simulink model "problem5"  (R2020b)
settings: Solver=VariableStepAuto  StartTime=0.0  StopTime=10.0  RelTol=1e-3
settings Model: Creator=Sourav Kumar  LastModifiedBy=Sourav Kumar

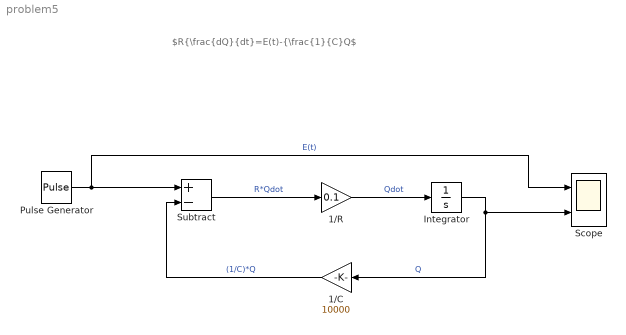
== system problem5 ==
  note: $R{\frac{dQ}{dt}=E(t)-{\frac{1}{C}Q$
  1/C : Gain  Gain=10000
  1/R : Gain  Gain=0.1
  Integrator : Integrator
  Pulse Generator : DiscretePulseGenerator  Amplitude=5
  Scope : Scope  NumInputPorts=2
  Subtract : Sum  Inputs=+-
  wires:
  Pulse Generator/1 -> Scope/1, Subtract/1  "E(t)"
  Subtract/1 -> 1/R/1  "R*Qdot"
  1/R/1 -> Integrator/1  "Qdot"
  Integrator/1 -> Scope/2, 1/C/1  "Q"
  1/C/1 -> Subtract/2  "(1/C)*Q"
